simulink model "simulation1_eeef366_5"  (R2017a)
settings: Solver=ode1  StartTime=0.0  StopTime=24*3600  FixedStep=60  MaxStep=60  RelTol=1e-3  EnableMultiTasking=on
InitFcn:
  | clc
  | tic
  | disp('----------------------------------')
  | disp(' ### Solving...')
  | disp('----------------------------------')
StartFcn:
  | disp(['Initialization took: ', num2str(toc), ' s'])
  | disp('Solving...')
  | tic
StopFcn:
  | dt = str2double(get_param([gcs, '/', 'powergui'], 'SampleTime'));
  | 
  | tend = str2double(get_param(gcs, 'StopTime'));
  | 
  | runTime = toc;
  | disp('----------------------------------')
  | disp(['### Simulation took: ', num2str(runTime), ' secs'])
  | 
  | disp(['### Simulation took: ', num2str(runTime/60), ' mins'])
  | 
  | numSteps = tend / dt;
  | 
  | disp(['### Steps / sec = ', num2str(numSteps / runTime)])
  | 
  | disp(['### Secs / step = ', num2str(runTime / numSteps)])
  | 
  | disp(['### Num. steps = ', num2str(numSteps)])
  | disp('----------------------------------')
libraries: powerlib x60, powerlib_extras x12, powerlib_meascontrol x1
(part 2 of 2)

== system simulation1_eeef366_5/Small Dynamic Load: Residential Microgrid/Smart Residential Complex/Distributed Generators for House01 ==
  Gain{1..3,5} (4 alike) : Gain  Gain=1e3
  "[IMPORT] Total House01 power consumption.csv" : FromWorkspace  VariableName=house01  OutputAfterFinalValue=Holding final value
      mask Display: image('C:\Users\Aryan Ritwajeet Jha\Desktop\CMS Desktop\3-2 2018-19\Mine\EEE F366\Foraged\Images\index.png');
  "[IMPORT] Total House01 power consumption.csv1" : FromWorkspace  VariableName=housepsolar01  OutputAfterFinalValue=Holding final value
      mask Display: image('C:\Users\Aryan Ritwajeet Jha\Desktop\CMS Desktop\3-2 2018-19\Mine\EEE F366\Foraged\Images\11.28_what-is-solar-energy.png');
  "[IMPORT] Total House01 power consumption.csv2" : FromWorkspace  VariableName=housepwind01  OutputAfterFinalValue=Holding final value
      mask Display: image('C:\Users\Aryan Ritwajeet Jha\Desktop\CMS Desktop\3-2 2018-19\Mine\EEE F366\Foraged\Images\647.jpg');
  "[IMPORT] Total House01 power consumption.csv3" : FromWorkspace  VariableName=housephouse01  OutputAfterFinalValue=Holding final value
      mask Display: image('C:\Users\Aryan Ritwajeet Jha\Desktop\CMS Desktop\3-2 2018-19\Mine\EEE F366\Foraged\Images\index.jpg');
  Out1 : Outport
  Out2 : Outport  Port=2
  Out3 : Outport  Port=3
  Out4 : Outport  Port=4
  wires:
  Gain3/1 -> Out4/1
  "[IMPORT] Total House01 power consumption.csv"/1 -> Gain3/1
  "[IMPORT] Total House01 power consumption.csv2"/1 -> Gain2/1
  "[IMPORT] Total House01 power consumption.csv1"/1 -> Gain1/1
  Gain5/1 -> Out1/1
  "[IMPORT] Total House01 power consumption.csv3"/1 -> Gain5/1
  Gain1/1 -> Out2/1
  Gain2/1 -> Out3/1

== system simulation1_eeef366_5/Small Dynamic Load: Residential Microgrid/Smart Residential Complex/Distributed Generators for House2 ==
  Gain{1..3,5} (4 alike) : Gain  Gain=1e3
  "[IMPORT] Total House01 power consumption.csv" : FromWorkspace  VariableName=house02  OutputAfterFinalValue=Holding final value
      mask Display: image('C:\Users\Aryan Ritwajeet Jha\Desktop\CMS Desktop\3-2 2018-19\Mine\EEE F366\Foraged\Images\index.png');
  "[IMPORT] Total House01 power consumption.csv1" : FromWorkspace  VariableName=housepsolar02  OutputAfterFinalValue=Holding final value
      mask Display: image('C:\Users\Aryan Ritwajeet Jha\Desktop\CMS Desktop\3-2 2018-19\Mine\EEE F366\Foraged\Images\11.28_what-is-solar-energy.png');
  "[IMPORT] Total House01 power consumption.csv2" : FromWorkspace  VariableName=housepwind02  OutputAfterFinalValue=Holding final value
      mask Display: image('C:\Users\Aryan Ritwajeet Jha\Desktop\CMS Desktop\3-2 2018-19\Mine\EEE F366\Foraged\Images\647.jpg');
  "[IMPORT] Total House01 power consumption.csv3" : FromWorkspace  VariableName=housephouse02  OutputAfterFinalValue=Holding final value
      mask Display: image('C:\Users\Aryan Ritwajeet Jha\Desktop\CMS Desktop\3-2 2018-19\Mine\EEE F366\Foraged\Images\index.jpg');
  Out1 : Outport
  Out2 : Outport  Port=2
  Out3 : Outport  Port=3
  Out4 : Outport  Port=4
  wires:
  Gain3/1 -> Out4/1
  "[IMPORT] Total House01 power consumption.csv"/1 -> Gain3/1
  "[IMPORT] Total House01 power consumption.csv2"/1 -> Gain2/1
  "[IMPORT] Total House01 power consumption.csv1"/1 -> Gain1/1
  Gain5/1 -> Out1/1
  "[IMPORT] Total House01 power consumption.csv3"/1 -> Gain5/1
  Gain1/1 -> Out2/1
  Gain2/1 -> Out3/1

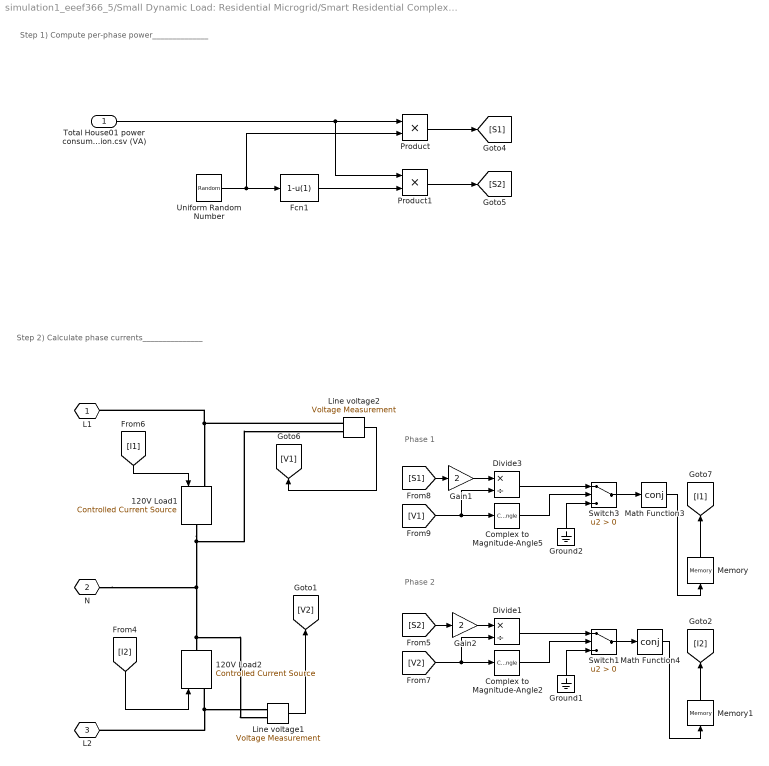
== system simulation1_eeef366_5/Small Dynamic Load: Residential Microgrid/Smart Residential Complex/House1 ==
  note: Phase 2
  note: Phase 1
  note: Step 2) Calculate phase currents_______________
  note: Step 1) Compute per-phase power______________
  Total House01 power consumption.csv (VA) : Inport
  120V Load1 : powerlib/Electrical Sources/Controlled Current Source  Initialize=off  Source_Type=AC  Amplitude=0  Phase=0  Frequency=0  Measurements=None
  120V Load2 : powerlib/Electrical Sources/Controlled Current Source  Initialize=off  Source_Type=AC  Amplitude=0  Phase=0  Frequency=0  Measurements=None
  Complex to Magnitude-Angle2 : ComplexToMagnitudeAngle  Output=Magnitude
  Complex to Magnitude-Angle5 : ComplexToMagnitudeAngle  Output=Magnitude
  Divide1 : Product  Inputs=*/
  Divide3 : Product  Inputs=*/
  Fcn1 : Fcn  Expr=1-u(1)
  Gain1 : Gain  Gain=2
  Gain2 : Gain  Gain=2
  Ground1 : Ground
  Ground2 : Ground
  Line voltage1 : powerlib/Measurements/Voltage Measurement  Tag=PoWeRsYsTeMmEaSuReMeNt  PhasorSimulation=on  OutputType=Complex  PSBequivalent=0
  Line voltage2 : powerlib/Measurements/Voltage Measurement  Tag=PoWeRsYsTeMmEaSuReMeNt  PhasorSimulation=on  OutputType=Complex  PSBequivalent=0
  Math Function3 : Math  Operator=conj  SaturateOnIntegerOverflow=on
  Math Function4 : Math  Operator=conj  SaturateOnIntegerOverflow=on
  Memory : Memory
  Memory1 : Memory
  Product : Product  RndMeth=Zero
  Product1 : Product  RndMeth=Zero
  Switch1 : Switch  Criteria=u2 > Threshold
  Switch3 : Switch  Criteria=u2 > Threshold
  Uniform Random Number : UniformRandomNumber  Minimum=0
  L1 : PMIOPort  Tag=PMCPort  Port=1  Side=Left
  N : PMIOPort  Tag=PMCPort  Port=2  Side=Left
  L2 : PMIOPort  Tag=PMCPort  Port=3  Side=Left
  wires:
  Total House01 power consumption.csv (VA)/1 -> Product/1, Product1/1
  Gain2/1 -> Divide1/1
  Gain1/1 -> Divide3/1
  Math Function4/1 -> Memory1/1
  Math Function3/1 -> Memory/1
  Fcn1/1 -> Product1/2
  Uniform Random Number/1 -> Fcn1/1, Product/2
  [I1] -> 120V Load1/1
  Switch1/1 -> Math Function4/1
  Ground1/1 -> Switch1/3
  Complex to Magnitude-Angle2/1 -> Switch1/2
  Divide1/1 -> Switch1/1
  [V2] -> Complex to Magnitude-Angle2/1, Divide1/2
  [S2] -> Gain2/1
  [I2] -> 120V Load2/1
  Line voltage1/1 -> [V2]
  Switch3/1 -> Math Function3/1
  Ground2/1 -> Switch3/3
  Complex to Magnitude-Angle5/1 -> Switch3/2
  Divide3/1 -> Switch3/1
  [V1] -> Divide3/2, Complex to Magnitude-Angle5/1
  [S1] -> Gain1/1
  Line voltage2/1 -> [V1]
  Product/1 -> [S1]
  Product1/1 -> [S2]
  Memory/1 -> [I1]
  Memory1/1 -> [I2]
  connections:
  L2/RConn1 -- Line voltage1/LConn1 -- 120V Load2/LConn1
  Line voltage2/LConn1 -- 120V Load1/LConn1 -- L1/RConn1
  N/RConn1 -- Line voltage1/LConn2 -- 120V Load2/RConn1 -- 120V Load1/RConn1 -- Line voltage2/LConn2

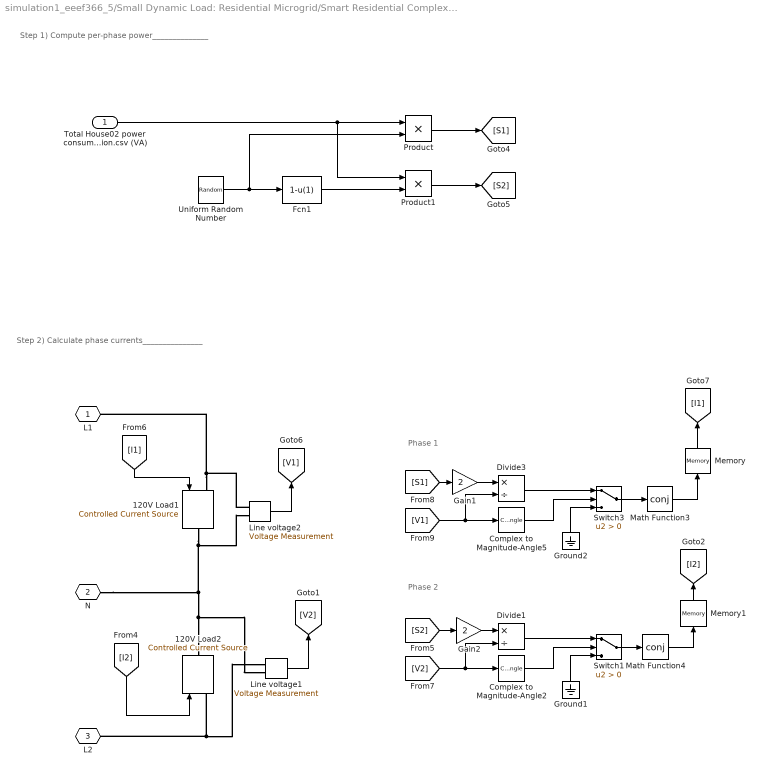
== system simulation1_eeef366_5/Small Dynamic Load: Residential Microgrid/Smart Residential Complex/House2 ==
  note: Step 1) Compute per-phase power______________
  note: Step 2) Calculate phase currents_______________
  note: Phase 1
  note: Phase 2
  Total House02 power consumption.csv (VA) : Inport
  120V Load1 : powerlib/Electrical Sources/Controlled Current Source  Initialize=off  Source_Type=AC  Amplitude=0  Phase=0  Frequency=0  Measurements=None
  120V Load2 : powerlib/Electrical Sources/Controlled Current Source  Initialize=off  Source_Type=AC  Amplitude=0  Phase=0  Frequency=0  Measurements=None
  Complex to Magnitude-Angle2 : ComplexToMagnitudeAngle  Output=Magnitude
  Complex to Magnitude-Angle5 : ComplexToMagnitudeAngle  Output=Magnitude
  Divide1 : Product  Inputs=*/
  Divide3 : Product  Inputs=*/
  Fcn1 : Fcn  Expr=1-u(1)
  Gain1 : Gain  Gain=2
  Gain2 : Gain  Gain=2
  Ground1 : Ground
  Ground2 : Ground
  Line voltage1 : powerlib/Measurements/Voltage Measurement  Tag=PoWeRsYsTeMmEaSuReMeNt  PhasorSimulation=on  OutputType=Complex  PSBequivalent=0
  Line voltage2 : powerlib/Measurements/Voltage Measurement  Tag=PoWeRsYsTeMmEaSuReMeNt  PhasorSimulation=on  OutputType=Complex  PSBequivalent=0
  Math Function3 : Math  Operator=conj  SaturateOnIntegerOverflow=on
  Math Function4 : Math  Operator=conj  SaturateOnIntegerOverflow=on
  Memory : Memory
  Memory1 : Memory
  Product : Product  RndMeth=Zero
  Product1 : Product  RndMeth=Zero
  Switch1 : Switch  Criteria=u2 > Threshold
  Switch3 : Switch  Criteria=u2 > Threshold
  Uniform Random Number : UniformRandomNumber  Minimum=0
  L1 : PMIOPort  Tag=PMCPort  Port=1  Side=Left
  N : PMIOPort  Tag=PMCPort  Port=2  Side=Left
  L2 : PMIOPort  Tag=PMCPort  Port=3  Side=Left
  wires:
  Memory1/1 -> [I2]
  Memory/1 -> [I1]
  Product1/1 -> [S2]
  Product/1 -> [S1]
  Line voltage2/1 -> [V1]
  [S1] -> Gain1/1
  [V1] -> Complex to Magnitude-Angle5/1, Divide3/2
  Divide3/1 -> Switch3/1
  Complex to Magnitude-Angle5/1 -> Switch3/2
  Ground2/1 -> Switch3/3
  Switch3/1 -> Math Function3/1
  Line voltage1/1 -> [V2]
  [I2] -> 120V Load2/1
  [S2] -> Gain2/1
  [V2] -> Divide1/2, Complex to Magnitude-Angle2/1
  Divide1/1 -> Switch1/1
  Complex to Magnitude-Angle2/1 -> Switch1/2
  Ground1/1 -> Switch1/3
  Switch1/1 -> Math Function4/1
  [I1] -> 120V Load1/1
  Uniform Random Number/1 -> Product/2, Fcn1/1
  Fcn1/1 -> Product1/2
  Math Function3/1 -> Memory/1
  Math Function4/1 -> Memory1/1
  Gain1/1 -> Divide3/1
  Gain2/1 -> Divide1/1
  Total House02 power consumption.csv (VA)/1 -> Product1/1, Product/1
  connections:
  120V Load1/LConn1 -- L1/RConn1 -- Line voltage2/LConn1
  120V Load2/LConn1 -- Line voltage1/LConn1 -- L2/RConn1
  N/RConn1 -- 120V Load1/RConn1 -- Line voltage2/LConn2 -- 120V Load2/RConn1 -- Line voltage1/LConn2

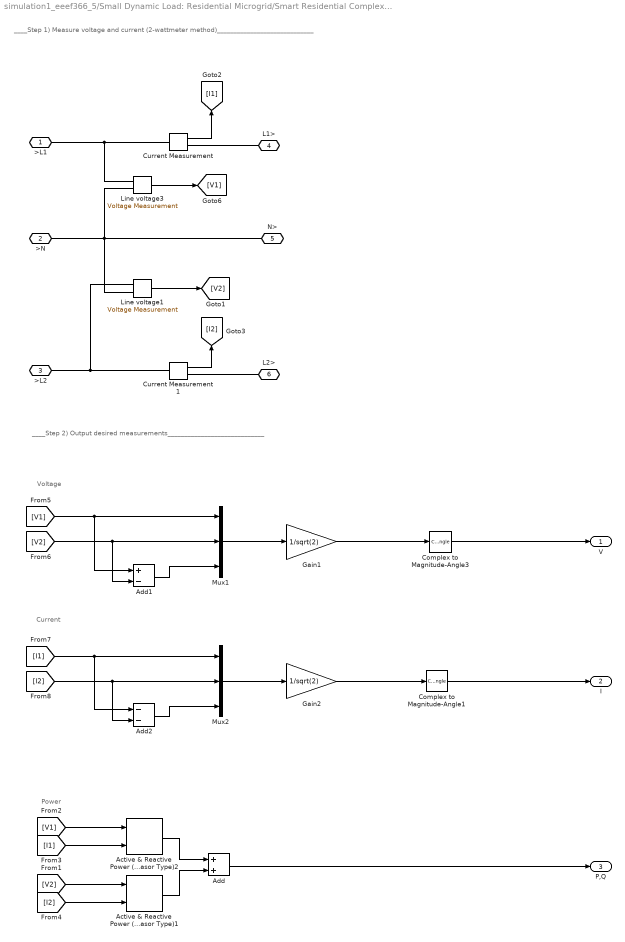
== system simulation1_eeef366_5/Small Dynamic Load: Residential Microgrid/Smart Residential Complex/Smart Meter House01 ==
  note: ____Step 1) Measure voltage and current (2-wattmeter method)_____________________________
  note: ____Step 2) Output desired measurements_____________________________
  note: Power
  note: Current
  note: Voltage
  Active & Reactive Power (Phasor Type)1 : powerlib_extras/Phasor Library/Active & Reactive Power (Phasor Type)
  Active & Reactive Power (Phasor Type)2 : powerlib_extras/Phasor Library/Active & Reactive Power (Phasor Type)
  Add : Sum
  Add1 : Sum  Inputs=+-
  Add2 : Sum  Inputs=--
  Complex to Magnitude-Angle1 : ComplexToMagnitudeAngle  Output=Magnitude
  Complex to Magnitude-Angle3 : ComplexToMagnitudeAngle  Output=Magnitude
  Current Measurement : powerlib/Measurements/Current Measurement  PhasorSimulation=on  OutputType=Complex  PSBequivalent=0
  Current Measurement1 : powerlib/Measurements/Current Measurement  PhasorSimulation=on  OutputType=Complex  PSBequivalent=0
  Gain1 : Gain  Gain=1/sqrt(2)
  Gain2 : Gain  Gain=1/sqrt(2)
  Line voltage1 : powerlib/Measurements/Voltage Measurement  Tag=PoWeRsYsTeMmEaSuReMeNt  PhasorSimulation=on  OutputType=Complex  PSBequivalent=0
  Line voltage3 : powerlib/Measurements/Voltage Measurement  Tag=PoWeRsYsTeMmEaSuReMeNt  PhasorSimulation=on  OutputType=Complex  PSBequivalent=0
  Mux1 : Mux  Inputs=3
  Mux2 : Mux  Inputs=3
  >L1 : PMIOPort  Port=1  Side=Left
      settings: AttributesFormatString=%<Side>
  >N : PMIOPort  Port=2  Side=Left
      settings: AttributesFormatString=%<Side>
  >L2 : PMIOPort  Port=3  Side=Left
      settings: AttributesFormatString=%<Side>
  L1> : PMIOPort  Port=4  Side=Right
      settings: AttributesFormatString=%<Side>
  N> : PMIOPort  Port=5  Side=Right
      settings: AttributesFormatString=%<Side>
  L2> : PMIOPort  Port=6  Side=Right
      settings: AttributesFormatString=%<Side>
  V : Outport
  I : Outport  Port=2
  P,Q : Outport  Port=3
  wires:
  Line voltage3/1 -> [V1]
  Line voltage1/1 -> [V2]
  Current Measurement/1 -> [I1]
  Current Measurement1/1 -> [I2]
  [V1] -> Active & Reactive Power (Phasor Type)2/1
  [I1] -> Active & Reactive Power (Phasor Type)2/2
  [V2] -> Active & Reactive Power (Phasor Type)1/1
  [I2] -> Active & Reactive Power (Phasor Type)1/2
  Active & Reactive Power (Phasor Type)2/1 -> Add/1
  Active & Reactive Power (Phasor Type)1/1 -> Add/2
  Add/1 -> P,Q/1
  [V1] -> Mux1/1, Add1/1
  [V2] -> Mux1/2, Add1/2
  Add1/1 -> Mux1/3
  Mux1/1 -> Gain1/1
  [I1] -> Add2/1, Mux2/1
  [I2] -> Add2/2, Mux2/2
  Add2/1 -> Mux2/3
  Mux2/1 -> Gain2/1
  Gain1/1 -> Complex to Magnitude-Angle3/1
  Gain2/1 -> Complex to Magnitude-Angle1/1
  Complex to Magnitude-Angle3/1 -> V/1
  Complex to Magnitude-Angle1/1 -> I/1
  connections:
  >L1/RConn1 -- Current Measurement/LConn1 -- Line voltage3/LConn1
  Current Measurement/RConn1 -- L1>/RConn1
  N>/RConn1 -- Line voltage3/LConn2 -- Line voltage1/LConn2 -- >N/RConn1
  >L2/RConn1 -- Line voltage1/LConn1 -- Current Measurement1/LConn1
  L2>/RConn1 -- Current Measurement1/RConn1

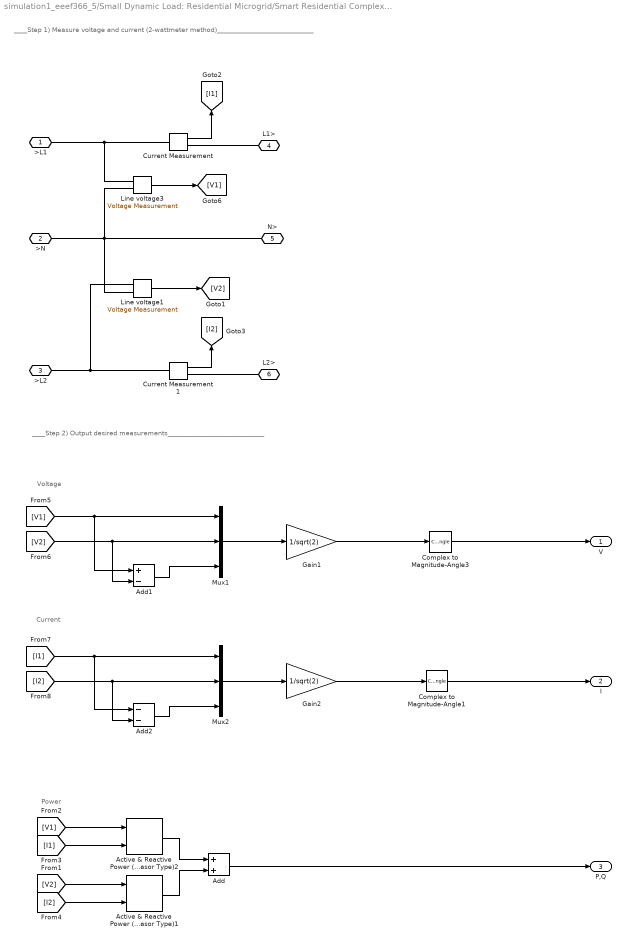
== system simulation1_eeef366_5/Small Dynamic Load: Residential Microgrid/Smart Residential Complex/Smart Meter House02 ==
  note: Voltage
  note: Current
  note: Power
  note: ____Step 2) Output desired measurements_____________________________
  note: ____Step 1) Measure voltage and current (2-wattmeter method)_____________________________
  Active & Reactive Power (Phasor Type)1 : powerlib_extras/Phasor Library/Active & Reactive Power (Phasor Type)
  Active & Reactive Power (Phasor Type)2 : powerlib_extras/Phasor Library/Active & Reactive Power (Phasor Type)
  Add : Sum
  Add1 : Sum  Inputs=+-
  Add2 : Sum  Inputs=--
  Complex to Magnitude-Angle1 : ComplexToMagnitudeAngle  Output=Magnitude
  Complex to Magnitude-Angle3 : ComplexToMagnitudeAngle  Output=Magnitude
  Current Measurement : powerlib/Measurements/Current Measurement  PhasorSimulation=on  OutputType=Complex  PSBequivalent=0
  Current Measurement1 : powerlib/Measurements/Current Measurement  PhasorSimulation=on  OutputType=Complex  PSBequivalent=0
  Gain1 : Gain  Gain=1/sqrt(2)
  Gain2 : Gain  Gain=1/sqrt(2)
  Line voltage1 : powerlib/Measurements/Voltage Measurement  Tag=PoWeRsYsTeMmEaSuReMeNt  PhasorSimulation=on  OutputType=Complex  PSBequivalent=0
  Line voltage3 : powerlib/Measurements/Voltage Measurement  Tag=PoWeRsYsTeMmEaSuReMeNt  PhasorSimulation=on  OutputType=Complex  PSBequivalent=0
  Mux1 : Mux  Inputs=3
  Mux2 : Mux  Inputs=3
  >L1 : PMIOPort  Port=1  Side=Left
      settings: AttributesFormatString=%<Side>
  >N : PMIOPort  Port=2  Side=Left
      settings: AttributesFormatString=%<Side>
  >L2 : PMIOPort  Port=3  Side=Left
      settings: AttributesFormatString=%<Side>
  L1> : PMIOPort  Port=4  Side=Right
      settings: AttributesFormatString=%<Side>
  N> : PMIOPort  Port=5  Side=Right
      settings: AttributesFormatString=%<Side>
  L2> : PMIOPort  Port=6  Side=Right
      settings: AttributesFormatString=%<Side>
  V : Outport
  I : Outport  Port=2
  P,Q : Outport  Port=3
  wires:
  Complex to Magnitude-Angle1/1 -> I/1
  Complex to Magnitude-Angle3/1 -> V/1
  Gain2/1 -> Complex to Magnitude-Angle1/1
  Gain1/1 -> Complex to Magnitude-Angle3/1
  Mux2/1 -> Gain2/1
  Add2/1 -> Mux2/3
  [I2] -> Mux2/2, Add2/2
  [I1] -> Mux2/1, Add2/1
  Mux1/1 -> Gain1/1
  Add1/1 -> Mux1/3
  [V2] -> Add1/2, Mux1/2
  [V1] -> Add1/1, Mux1/1
  Add/1 -> P,Q/1
  Active & Reactive Power (Phasor Type)1/1 -> Add/2
  Active & Reactive Power (Phasor Type)2/1 -> Add/1
  [I2] -> Active & Reactive Power (Phasor Type)1/2
  [V2] -> Active & Reactive Power (Phasor Type)1/1
  [I1] -> Active & Reactive Power (Phasor Type)2/2
  [V1] -> Active & Reactive Power (Phasor Type)2/1
  Current Measurement1/1 -> [I2]
  Current Measurement/1 -> [I1]
  Line voltage1/1 -> [V2]
  Line voltage3/1 -> [V1]
  connections:
  L2>/RConn1 -- Current Measurement1/RConn1
  Line voltage1/LConn1 -- >L2/RConn1 -- Current Measurement1/LConn1
  Line voltage3/LConn2 -- N>/RConn1 -- >N/RConn1 -- Line voltage1/LConn2
  Current Measurement/RConn1 -- L1>/RConn1
  Current Measurement/LConn1 -- >L1/RConn1 -- Line voltage3/LConn1
